simulink model "SetPlanning"  (R2019b)
settings: Solver=FixedStepAuto  StartTime=0.0  StopTime=1.5  FixedStep=0.001  RelTol=1e-5
libraries: cstblocks x3, simulink x2
settings Model: PacingRate=0.032000  Creator=lenovo  LastModifiedBy=lenovo

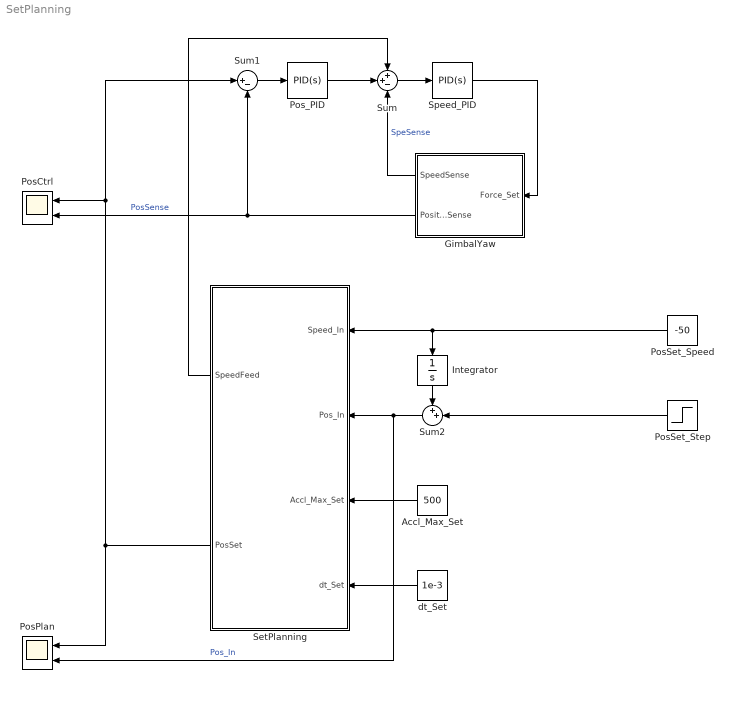
== system SetPlanning ==
  Accl_Max_Set : Constant  Value=500
  GimbalYaw : Subsystem
  Integrator : Integrator
  PosCtrl : Scope  NumInputPorts=2
  PosPlan : Scope  NumInputPorts=2
  PosSet_Speed : Constant  Value=-50
  PosSet_Step : Step  Time=0.5  After=90  SampleTime=0
  Pos_PID : simulink/Continuous/PID Controller  Controller=PID  Form=Parallel  TimeDomain=Continuous-time  SampleTime=-1  IntegratorMethod=Forward Euler  FilterMethod=Forward Euler  ControllerParametersSource=internal  P=45  I=0  D=1.8  UseFilter=on  N=100  TunerSelectOption=Transfer Function Based (PID Tuner App)  InitialConditionSource=internal  InitialConditionForIntegrator=0  InitialConditionForFilter=0  DifferentiatorICPrevScaledInput=0  ExternalReset=none  TrackingMode=off  Kt=1  LimitOutput=off  UpperSaturationLimit=inf  LowerSaturationLimit=-inf  LinearizeAsGain=on  AntiWindupMode=none  Kb=1  POutMin=[]  POutMax=[]  IOutMin=[]  IOutMax=[]  DOutMin=[]  DOutMax=[]  NOutMin=[]  NOutMax=[]  SumOutMin=[]  SumOutMax=[]  SaturationOutMin=[]  SaturationOutMax=[]  PParamMin=[]  PParamMax=[]  IParamMin=[]  IParamMax=[]  DParamMin=[]  DParamMax=[]  NParamMin=[]  NParamMax=[]  KbParamMin=[]  KbParamMax=[]  KtParamMin=[]  KtParamMax=[]  KbOutMin=[]  KbOutMax=[]  KtOutMin=[]  KtOutMax=[]  IntegratorOutMin=[]  IntegratorOutMax=[]  FilterOutMin=[]  FilterOutMax=[]  SumI1OutMin=[]  SumI1OutMax=[]  SumI2OutMin=[]  SumI2OutMax=[]  SumI3OutMin=[]  SumI3OutMax=[]  SumI4OutMin=[]  SumI4OutMax=[]  SumDOutMin=[]  SumDOutMax=[]  DifferentiatorOutMin=[]  DifferentiatorOutMax=[]  FilterDiffOutCoefMin=[]  FilterDiffOutCoefMax=[]  ReciprocalOutMin=[]  ReciprocalOutMax=[]  SumDenOutMin=[]  SumDenOutMax=[]  SumNumOutMin=[]  SumNumOutMax=[]  DivideOutMin=[]  DivideOutMax=[]  IntegratorContinuousStateAttributes=''  IntegratorStateMustResolveToSignalObject=off  IntegratorRTWStateStorageClass=Auto  FilterContinuousStateAttributes=''  FilterStateMustResolveToSignalObject=off  FilterRTWStateStorageClass=Auto  ParallelPVariant=InternalParameters  IdealPVariant=Disabled  IVariant=InternalParameters  DVariant=InternalParameters  IntegratorVariant=Continuous  SatVariant=Disabled  AWVariant=Passthrough  PCopyVariant=Disabled  TRVariant=Disabled  FdbkBlocksVariant=Forward  IdealPFdbkVariant=Disabled  SatFdbkVariant=Disabled  DerivativeFilterVariant=ContFilter  NVariant=InternalParameters  NCopyVariant=Disabled  FilterICVariant=InternalICsFilter  IntegratorICVariant=InternalICs  ExternalResetVariant=Disabled  TRSumVariant=Passthrough  SumFdbkVariant=Disabled  SumVariant=Sum_PID
  SetPlanning : Subsystem
  Speed_PID : simulink/Continuous/PID Controller  Controller=PID  Form=Parallel  TimeDomain=Continuous-time  SampleTime=-1  IntegratorMethod=Forward Euler  FilterMethod=Forward Euler  ControllerParametersSource=internal  P=150  I=5  D=0.5  UseFilter=on  N=100  TunerSelectOption=Transfer Function Based (PID Tuner App)  InitialConditionSource=internal  InitialConditionForIntegrator=0  InitialConditionForFilter=0  DifferentiatorICPrevScaledInput=0  ExternalReset=none  TrackingMode=off  Kt=1  LimitOutput=off  UpperSaturationLimit=inf  LowerSaturationLimit=-inf  LinearizeAsGain=on  AntiWindupMode=none  Kb=1  POutMin=[]  POutMax=[]  IOutMin=[]  IOutMax=[]  DOutMin=[]  DOutMax=[]  NOutMin=[]  NOutMax=[]  SumOutMin=[]  SumOutMax=[]  SaturationOutMin=[]  SaturationOutMax=[]  PParamMin=[]  PParamMax=[]  IParamMin=[]  IParamMax=[]  DParamMin=[]  DParamMax=[]  NParamMin=[]  NParamMax=[]  KbParamMin=[]  KbParamMax=[]  KtParamMin=[]  KtParamMax=[]  KbOutMin=[]  KbOutMax=[]  KtOutMin=[]  KtOutMax=[]  IntegratorOutMin=[]  IntegratorOutMax=[]  FilterOutMin=[]  FilterOutMax=[]  SumI1OutMin=[]  SumI1OutMax=[]  SumI2OutMin=[]  SumI2OutMax=[]  SumI3OutMin=[]  SumI3OutMax=[]  SumI4OutMin=[]  SumI4OutMax=[]  SumDOutMin=[]  SumDOutMax=[]  DifferentiatorOutMin=[]  DifferentiatorOutMax=[]  FilterDiffOutCoefMin=[]  FilterDiffOutCoefMax=[]  ReciprocalOutMin=[]  ReciprocalOutMax=[]  SumDenOutMin=[]  SumDenOutMax=[]  SumNumOutMin=[]  SumNumOutMax=[]  DivideOutMin=[]  DivideOutMax=[]  IntegratorContinuousStateAttributes=''  IntegratorStateMustResolveToSignalObject=off  IntegratorRTWStateStorageClass=Auto  FilterContinuousStateAttributes=''  FilterStateMustResolveToSignalObject=off  FilterRTWStateStorageClass=Auto  ParallelPVariant=InternalParameters  IdealPVariant=Disabled  IVariant=InternalParameters  DVariant=InternalParameters  IntegratorVariant=Continuous  SatVariant=Disabled  AWVariant=Passthrough  PCopyVariant=Disabled  TRVariant=Disabled  FdbkBlocksVariant=Forward  IdealPFdbkVariant=Disabled  SatFdbkVariant=Disabled  DerivativeFilterVariant=ContFilter  NVariant=InternalParameters  NCopyVariant=Disabled  FilterICVariant=InternalICsFilter  IntegratorICVariant=InternalICs  ExternalResetVariant=Disabled  TRSumVariant=Passthrough  SumFdbkVariant=Disabled  SumVariant=Sum_PID
  Sum : Sum  Inputs=++-
  Sum1 : Sum  Inputs=|+-
  Sum2 : Sum  Inputs=++|
  dt_Set : Constant  Value=1e-3
  wires:
  Sum/1 -> Speed_PID/1
  GimbalYaw/1(SpeedSense) -> Sum/3  "SpeSense"
  Speed_PID/1 -> GimbalYaw/1(Force_Set)
  Pos_PID/1 -> Sum/2
  Sum1/1 -> Pos_PID/1
  GimbalYaw/2(PositonSense) -> Sum1/2, PosCtrl/2  "PosSense"
  PosSet_Step/1 -> Sum2/2
  Accl_Max_Set/1 -> SetPlanning/3(Accl_Max_Set)
  dt_Set/1 -> SetPlanning/4(dt_Set)
  SetPlanning/1(SpeedFeed) -> Sum/1
  SetPlanning/2(PosSet) -> Sum1/1, PosCtrl/1, PosPlan/1
  Sum2/1 -> PosPlan/2, SetPlanning/2(Pos_In)  "Pos_In"
  Integrator/1 -> Sum2/1
  PosSet_Speed/1 -> SetPlanning/1(Speed_In), Integrator/1

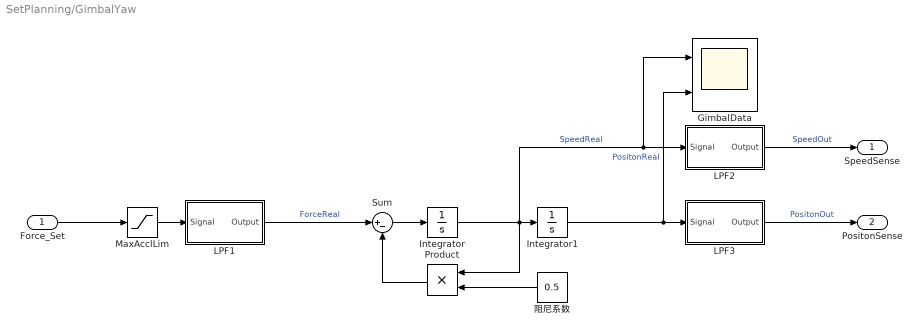
== system SetPlanning/GimbalYaw ==
  Force_Set : Inport
  GimbalData : Scope  NumInputPorts=2
  Integrator : Integrator
  Integrator1 : Integrator
  LPF1 : Subsystem  mask{Frq=400}
      mask prompts: Frq "Frq_Set"
  LPF2 : Subsystem  mask{Frq=800}
      mask prompts: Frq "Frq_Set"
  LPF3 : Subsystem  mask{Frq=800}
      mask prompts: Frq "Frq_Set"
  MaxAcclLim : Saturate  UpperLimit=800  LowerLimit=-800
  Product : Product
  Sum : Sum  Inputs=|+-
  阻尼系数 : Constant  Value=0.5
  SpeedSense : Outport
  PositonSense : Outport  Port=2
  wires:
  Product/1 -> Sum/2
  Sum/1 -> Integrator/1
  Integrator/1 -> GimbalData/1, LPF2/1(Signal), Product/1, Integrator1/1  "SpeedReal"
  阻尼系数/1 -> Product/2
  Force_Set/1 -> MaxAcclLim/1
  Integrator1/1 -> GimbalData/2, LPF3/1(Signal)  "PositonReal"
  MaxAcclLim/1 -> LPF1/1(Signal)
  LPF1/1(Output) -> Sum/1  "ForceReal"
  LPF2/1(Output) -> SpeedSense/1  "SpeedOut"
  LPF3/1(Output) -> PositonSense/1  "PositonOut"

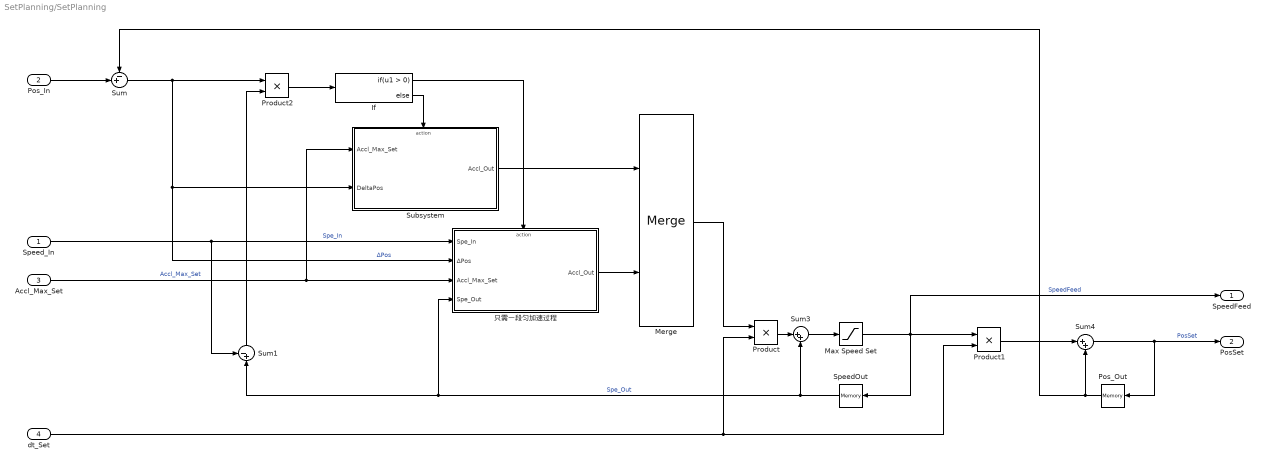
== system SetPlanning/SetPlanning ==
  Speed_In : Inport
  Pos_In : Inport  Port=2
  Accl_Max_Set : Inport  Port=3
  dt_Set : Inport  Port=4
  If : If
  Max Speed Set : Saturate  UpperLimit=300  LowerLimit=-300
  Merge : Merge
  Pos_Out : Memory
  Product : Product
  Product1 : Product
  Product2 : Product
  SpeedOut : Memory
  Subsystem : Subsystem
  Sum : Sum  Inputs=-+|
  Sum1 : Sum  Inputs=-+|
  Sum3 : Sum  Inputs=|++
  Sum4 : Sum  Inputs=|++
  只需一段匀加速过程 : Subsystem
  SpeedFeed : Outport
  PosSet : Outport  Port=2
  wires:
  Sum4/1 -> PosSet/1, Pos_Out/1  "PosSet"
  SpeedOut/1 -> 只需一段匀加速过程/4(Spe_Out), Sum1/2, Sum3/2  "Spe_Out"
  Sum3/1 -> Max Speed Set/1
  Max Speed Set/1 -> Product1/1, SpeedFeed/1, SpeedOut/1  "SpeedFeed"
  Pos_Out/1 -> Sum/1, Sum4/2
  Product/1 -> Sum3/1
  Product1/1 -> Sum4/1
  dt_Set/1 -> Product/2, Product1/2
  Pos_In/1 -> Sum/2
  Speed_In/1 -> Sum1/1, 只需一段匀加速过程/1(Spe_In)  "Spe_In"
  Sum/1 -> Subsystem/2(DeltaPos), 只需一段匀加速过程/2(ΔPos), Product2/1  "ΔPos"
  Accl_Max_Set/1 -> Subsystem/1(Accl_Max_Set), 只需一段匀加速过程/3(Accl_Max_Set)  "Accl_Max_Set"
  Product2/1 -> If/1
  If/1 -> 只需一段匀加速过程/Action
  Subsystem/1(Accl_Out) -> Merge/1
  If/2 -> Subsystem/Action
  只需一段匀加速过程/1(Accl_Out) -> Merge/2
  Merge/1 -> Product/1
  Sum1/1 -> Product2/2

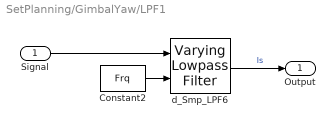
== system SetPlanning/GimbalYaw/LPF1 ==
  Signal : Inport
  Constant2 : Constant  Value=Frq
  d_Smp_LPF6 : cstblocks/Linear Parameter Varying/Varying Lowpass Filter  N=1
      settings: SourceProductName=Control System Toolbox
  Output : Outport
  wires:
  d_Smp_LPF6/1 -> Output/1  "Is"
  Constant2/1 -> d_Smp_LPF6/2
  Signal/1 -> d_Smp_LPF6/1

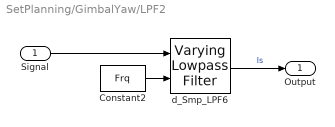
== system SetPlanning/GimbalYaw/LPF2 ==
  Signal : Inport
  Constant2 : Constant  Value=Frq
  d_Smp_LPF6 : cstblocks/Linear Parameter Varying/Varying Lowpass Filter  N=1
      settings: SourceProductName=Control System Toolbox
  Output : Outport
  wires:
  d_Smp_LPF6/1 -> Output/1  "Is"
  Constant2/1 -> d_Smp_LPF6/2
  Signal/1 -> d_Smp_LPF6/1

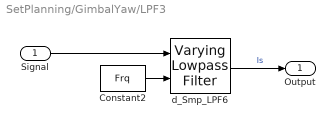
== system SetPlanning/GimbalYaw/LPF3 ==
  Signal : Inport
  Constant2 : Constant  Value=Frq
  d_Smp_LPF6 : cstblocks/Linear Parameter Varying/Varying Lowpass Filter  N=1
      settings: SourceProductName=Control System Toolbox
  Output : Outport
  wires:
  d_Smp_LPF6/1 -> Output/1  "Is"
  Constant2/1 -> d_Smp_LPF6/2
  Signal/1 -> d_Smp_LPF6/1

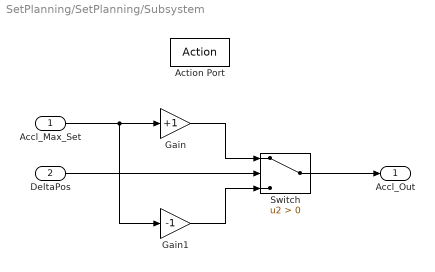
== system SetPlanning/SetPlanning/Subsystem ==
  Accl_Max_Set : Inport
  DeltaPos : Inport  Port=2
  Action Port : ActionPort  ActionPortLabel=else
  Gain : Gain  Gain=+1
  Gain1 : Gain  Gain=-1
  Switch : Switch  Criteria=u2 > Threshold
  Accl_Out : Outport
  wires:
  Accl_Max_Set/1 -> Gain1/1, Gain/1
  Switch/1 -> Accl_Out/1
  Gain/1 -> Switch/1
  DeltaPos/1 -> Switch/2
  Gain1/1 -> Switch/3

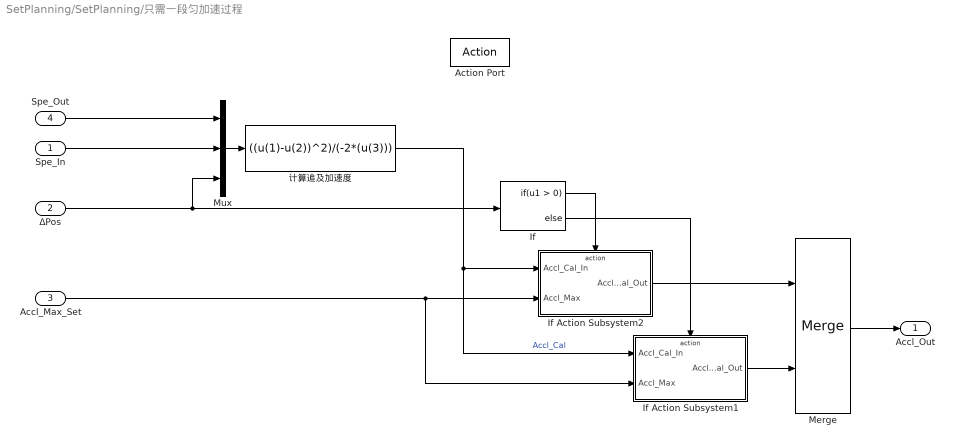
== system SetPlanning/SetPlanning/只需一段匀加速过程 ==
  Spe_In : Inport
  ΔPos : Inport  Port=2
  Accl_Max_Set : Inport  Port=3
  Spe_Out : Inport  Port=4
  Action Port : ActionPort  ActionPortLabel=if(u1 > 0)
  If : If
  If Action Subsystem1 : Subsystem  TreatAsAtomicUnit=on
  If Action Subsystem2 : Subsystem  TreatAsAtomicUnit=on
  Merge : Merge
  Mux : Mux  Inputs=3
  计算追及加速度 : Fcn  Expr=((u(1)-u(2))^2)/(-2*(u(3)))
  Accl_Out : Outport
  wires:
  Mux/1 -> 计算追及加速度/1
  Accl_Max_Set/1 -> If Action Subsystem1/2(Accl_Max), If Action Subsystem2/2(Accl_Max)
  计算追及加速度/1 -> If Action Subsystem1/1(Accl_Cal_In), If Action Subsystem2/1(Accl_Cal_In)  "Accl_Cal"
  If Action Subsystem1/1(Accl_Cal_Out) -> Merge/2
  If/1 -> If Action Subsystem2/Action
  Spe_In/1 -> Mux/2
  ΔPos/1 -> Mux/3, If/1
  If/2 -> If Action Subsystem1/Action
  If Action Subsystem2/1(Accl_Cal_Out) -> Merge/1
  Spe_Out/1 -> Mux/1
  Merge/1 -> Accl_Out/1

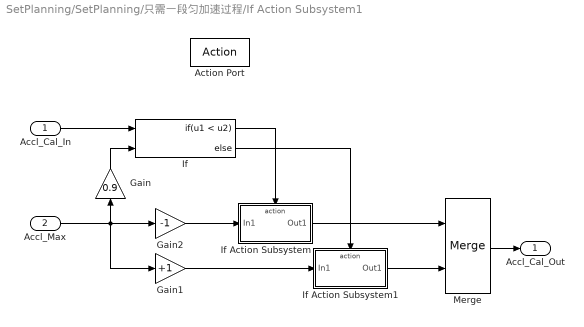
== system SetPlanning/SetPlanning/只需一段匀加速过程/If Action Subsystem1 ==
  Accl_Cal_In : Inport
  Accl_Max : Inport  Port=2
  Action Port : ActionPort  ActionPortLabel=else
  Gain : Gain  Gain=0.9
  Gain1 : Gain  Gain=+1
  Gain2 : Gain  Gain=-1
  If : If  NumInputs=2  IfExpression=u1 < u2
  If Action Subsystem : Subsystem  TreatAsAtomicUnit=on
  If Action Subsystem1 : Subsystem  TreatAsAtomicUnit=on
  Merge : Merge
  Accl_Cal_Out : Outport
  wires:
  Gain/1 -> If/2
  If Action Subsystem/1(Out1) -> Merge/1
  If/1 -> If Action Subsystem/Action
  Accl_Max/1 -> Gain1/1, Gain2/1, Gain/1
  If Action Subsystem1/1(Out1) -> Merge/2
  Accl_Cal_In/1 -> If/1
  If/2 -> If Action Subsystem1/Action
  Gain1/1 -> If Action Subsystem1/1(In1)
  Merge/1 -> Accl_Cal_Out/1
  Gain2/1 -> If Action Subsystem/1(In1)

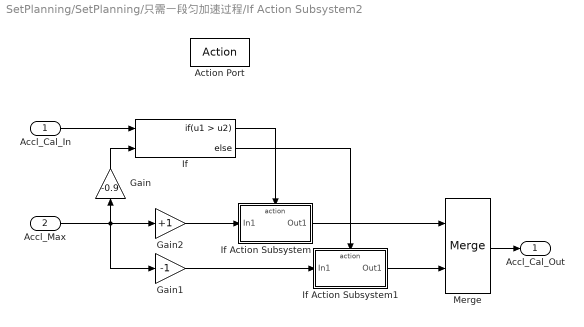
== system SetPlanning/SetPlanning/只需一段匀加速过程/If Action Subsystem2 ==
  Accl_Cal_In : Inport
  Accl_Max : Inport  Port=2
  Action Port : ActionPort  ActionPortLabel=if(u1 > 0)
  Gain : Gain  Gain=-0.9
  Gain1 : Gain  Gain=-1
  Gain2 : Gain  Gain=+1
  If : If  NumInputs=2  IfExpression=u1 > u2
  If Action Subsystem : Subsystem  TreatAsAtomicUnit=on
  If Action Subsystem1 : Subsystem  TreatAsAtomicUnit=on
  Merge : Merge
  Accl_Cal_Out : Outport
  wires:
  Gain/1 -> If/2
  If Action Subsystem/1(Out1) -> Merge/1
  If/1 -> If Action Subsystem/Action
  Accl_Max/1 -> Gain1/1, Gain2/1, Gain/1
  If Action Subsystem1/1(Out1) -> Merge/2
  Accl_Cal_In/1 -> If/1
  If/2 -> If Action Subsystem1/Action
  Gain1/1 -> If Action Subsystem1/1(In1)
  Merge/1 -> Accl_Cal_Out/1
  Gain2/1 -> If Action Subsystem/1(In1)

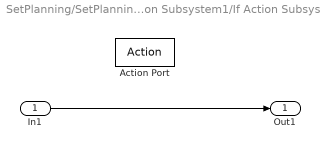
== system SetPlanning/SetPlanning/只需一段匀加速过程/If Action Subsystem1/If Action Subsystem ==
  In1 : Inport
  Action Port : ActionPort  ActionPortLabel=if(u1 < u2)
  Out1 : Outport
  wires:
  In1/1 -> Out1/1

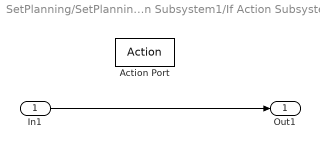
== system SetPlanning/SetPlanning/只需一段匀加速过程/If Action Subsystem1/If Action Subsystem1 ==
  In1 : Inport
  Action Port : ActionPort  ActionPortLabel=else
  Out1 : Outport
  wires:
  In1/1 -> Out1/1

== system SetPlanning/SetPlanning/只需一段匀加速过程/If Action Subsystem2/If Action Subsystem ==
  In1 : Inport
  Action Port : ActionPort  ActionPortLabel=if(u1 > u2)
  Out1 : Outport
  wires:
  In1/1 -> Out1/1

== system SetPlanning/SetPlanning/只需一段匀加速过程/If Action Subsystem2/If Action Subsystem1 ==
  In1 : Inport
  Action Port : ActionPort  ActionPortLabel=else
  Out1 : Outport
  wires:
  In1/1 -> Out1/1
